simulink model "testI2tSineInput"  (R2016b)
settings: Solver=FixedStepAuto  StartTime=0.0  StopTime=180  FixedStep=0.002  RelTol=1e-3
libraries: I2t x1
settings Model: DataDictionary=ModelDictionary.sldd  Creator=Marc  LastModifiedBy=Marc
settings DataIOCC: ExternalInput=a

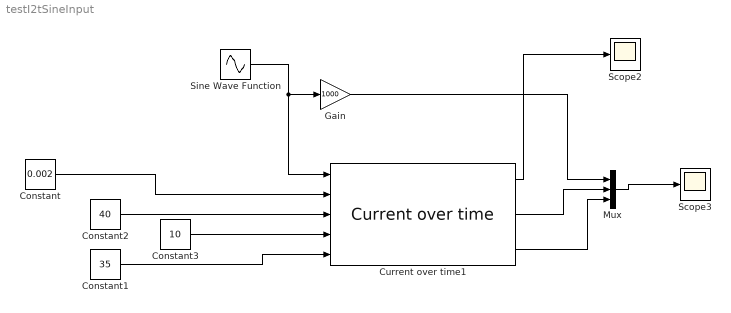
== system testI2tSineInput ==
  Constant : Constant  Value=0.002
  Constant1 : Constant  Value=35
  Constant2 : Constant  Value=40
  Constant3 : Constant  Value=10
  Current over time1 : I2t/Current over time
  Gain : Gain  Gain=1000
  Mux : Mux  Inputs=3
  Scope2 : Scope
  Scope3 : Scope
  Sine Wave Function : Sin  SineType=Sample based  Amplitude=18  Bias=20  Samples=15000  SampleTime=0.002
  wires:
  Current over time1/1 -> Scope2/1
  Mux/1 -> Scope3/1
  Constant/1 -> Current over time1/2
  Current over time1/2 -> Mux/2
  Current over time1/3 -> Mux/3
  Constant3/1 -> Current over time1/4
  Constant2/1 -> Current over time1/3
  Constant1/1 -> Current over time1/5
  Sine Wave Function/1 -> Gain/1, Current over time1/1
  Gain/1 -> Mux/1
